simulink model "obs5_simulink"  (R2020b)
settings: Solver=VariableStepAuto  StartTime=0.0  StopTime=0  RelTol=1e-3
settings Model: Creator=Mohit Akhouri  LastModifiedBy=Mohit Akhouri

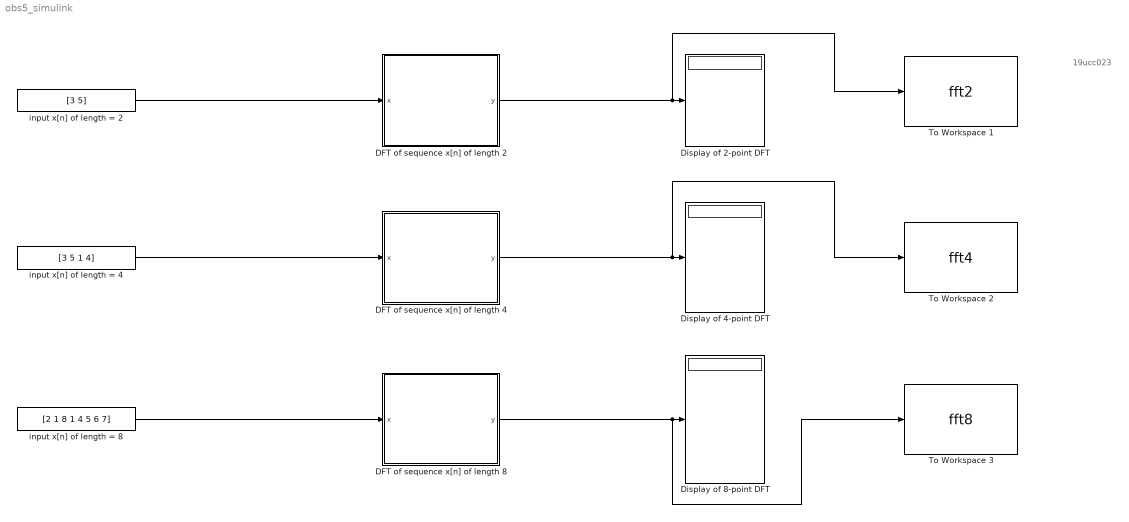
== system obs5_simulink ==
  note: 19ucc023
  DFT of sequence x[n] of length 2 : MATLAB Function  TreatAsAtomicUnit=on
  DFT of sequence x[n] of length 4 : MATLAB Function  TreatAsAtomicUnit=on
  DFT of sequence x[n] of length 8 : MATLAB Function  TreatAsAtomicUnit=on
  Display of 2-point DFT : Display
  Display of 4-point DFT : Display
  Display of 8-point DFT : Display
  To Workspace 1 : ToWorkspace  VariableName=fft2  SaveFormat=Timeseries  SampleTime=-1
  To Workspace 2 : ToWorkspace  VariableName=fft4  SaveFormat=Timeseries  SampleTime=-1
  To Workspace 3 : ToWorkspace  VariableName=fft8  SaveFormat=Timeseries  SampleTime=-1
  input x[n] of length = 2 : Constant  Value=[3 5]
  input x[n] of length = 4 : Constant  Value=[3 5 1 4]
  input x[n] of length = 8 : Constant  Value=[2 1 8 1 4 5 6 7]
  wires:
  input x[n] of length = 2/1 -> DFT of sequence x[n] of length 2/1(x)
  input x[n] of length = 4/1 -> DFT of sequence x[n] of length 4/1(x)
  input x[n] of length = 8/1 -> DFT of sequence x[n] of length 8/1(x)
  DFT of sequence x[n] of length 2/1(y) -> To Workspace 1/1, Display of 2-point DFT/1
  DFT of sequence x[n] of length 4/1(y) -> To Workspace 2/1, Display of 4-point DFT/1
  DFT of sequence x[n] of length 8/1(y) -> To Workspace 3/1, Display of 8-point DFT/1

== matlab function obs5_simulink/DFT of sequence x[n] of length 2 ==
  data: x input; y output
function y = fcn(x)
% This function will calculate DFT of sequence x[n] of length N via radix-2
% fft algorithm

N = length(x);
y = complex(zeros(1,N)); % Output variable to store N-point DFT

% Adjusting the sequence x[n] to make its length equivalent to 'power of 2'

length_x = length(x); % length of sequence x[n]
ind = log(length_x)/log(2); % taking log to determine the index
ind = ceil(ind); % taking ceil function to make 'ind' a integer value
size_adj = 2^ind; % calculated length in powers of 2

x = [x zeros(1,size_adj-length_x)]; % adjusting x[n] by adding zeros 

f1 = complex(zeros(1,N/2)); % to store the DFT of ODD parts of x[n]
f2 = complex(zeros(1,N/2)); % to store the DFT of EVEN parts of x[n]
Wn = exp(-1j*2*pi/N); % twiddle factor used in calculation of DFT

% Loop for calculation of DFT via radix-2 fft method
for k=1:N/2
    for m=1:N/2
        f1(k) = f1(k) + (x(2*(m-1)+1)*(Wn^(2*(m-1)*(k-1))));
        f2(k) = f2(k) + (x(2*(m-1)+2)*(Wn^(2*(m-1)*(k-1))));
    end
    y(k) = f1(k) + f2(k)*(Wn^(k-1)); % First half of DFT of sequence x[n]
    y(k+N/2) = f1(k) - f2(k)*(Wn^(k-1)); % Second half of DFT of sequence x[n]
end

== matlab function obs5_simulink/DFT of sequence x[n] of length 8 ==
  data: x input; y output
function y = fcn(x)
% This function will calculate DFT of sequence x[n] of length N via radix-2
% fft algorithm

N = length(x);
y = complex(zeros(1,N)); % Output variable to store N-point DFT

% Adjusting the sequence x[n] to make its length equivalent to 'power of 2'

length_x = length(x); % length of sequence x[n]
ind = log(length_x)/log(2); % taking log to determine the index
ind = ceil(ind); % taking ceil function to make 'ind' a integer value
size_adj = 2^ind; % calculated length in powers of 2

x = [x zeros(1,size_adj-length_x)]; % adjusting x[n] by adding zeros 

f1 = complex(zeros(1,N/2)); % to store the DFT of ODD parts of x[n]
f2 = complex(zeros(1,N/2)); % to store the DFT of EVEN parts of x[n]
Wn = exp(-1j*2*pi/N); % twiddle factor used in calculation of DFT

% Loop for calculation of DFT via radix-2 fft method
for k=1:N/2
    for m=1:N/2
        f1(k) = f1(k) + (x(2*(m-1)+1)*(Wn^(2*(m-1)*(k-1))));
        f2(k) = f2(k) + (x(2*(m-1)+2)*(Wn^(2*(m-1)*(k-1))));
    end
    y(k) = f1(k) + f2(k)*(Wn^(k-1)); % First half of DFT of sequence x[n]
    y(k+N/2) = f1(k) - f2(k)*(Wn^(k-1)); % Second half of DFT of sequence x[n]
end

== matlab function obs5_simulink/DFT of sequence x[n] of length 4 ==
  data: x input; y output
function y = fcn(x)
% This function will calculate DFT of sequence x[n] of length N via radix-2
% fft algorithm

N = length(x);
y = complex(zeros(1,N)); % Output variable to store N-point DFT

% Adjusting the sequence x[n] to make its length equivalent to 'power of 2'

length_x = length(x); % length of sequence x[n]
ind = log(length_x)/log(2); % taking log to determine the index
ind = ceil(ind); % taking ceil function to make 'ind' a integer value
size_adj = 2^ind; % calculated length in powers of 2

x = [x zeros(1,size_adj-length_x)]; % adjusting x[n] by adding zeros 

f1 = complex(zeros(1,N/2)); % to store the DFT of ODD parts of x[n]
f2 = complex(zeros(1,N/2)); % to store the DFT of EVEN parts of x[n]
Wn = exp(-1j*2*pi/N); % twiddle factor used in calculation of DFT

% Loop for calculation of DFT via radix-2 fft method
for k=1:N/2
    for m=1:N/2
        f1(k) = f1(k) + (x(2*(m-1)+1)*(Wn^(2*(m-1)*(k-1))));
        f2(k) = f2(k) + (x(2*(m-1)+2)*(Wn^(2*(m-1)*(k-1))));
    end
    y(k) = f1(k) + f2(k)*(Wn^(k-1)); % First half of DFT of sequence x[n]
    y(k+N/2) = f1(k) - f2(k)*(Wn^(k-1)); % Second half of DFT of sequence x[n]
end
